simulink model "Parabolic_Shooting_exercise"  (R2020b)
settings: Solver=VariableStepAuto  StartTime=0.0  StopTime=inf  RelTol=1e-3
settings Model: Creator=gbellido  LastModifiedBy=gbellido

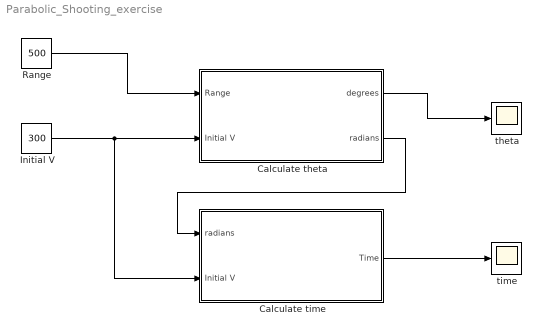
== system Parabolic_Shooting_exercise ==
  Calculate theta : Subsystem
  Calculate time : Subsystem
  Initial V : Constant  Value=300
  Range : Constant  Value=500
  theta : Scope
  time : Scope
  wires:
  Initial V/1 -> Calculate time/2(Initial V), Calculate theta/2(Initial V)
  Calculate theta/1(degrees) -> theta/1
  Calculate time/1(Time) -> time/1
  Calculate theta/2(radians) -> Calculate time/1(radians)
  Range/1 -> Calculate theta/1(Range)

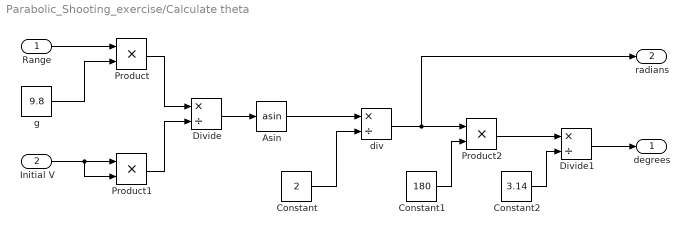
== system Parabolic_Shooting_exercise/Calculate theta ==
  Range : Inport
  Initial V : Inport  Port=2
  Asin : Trigonometry  Operator=asin
  Constant : Constant  Value=2
  Constant1 : Constant  Value=180
  Constant2 : Constant  Value=3.14
  Divide : Product  Inputs=*/
  Divide1 : Product  Inputs=*/
  Product : Product
  Product1 : Product
  Product2 : Product
  div : Product  Inputs=*/
  g : Constant  Value=9.8
  degrees : Outport
  radians : Outport  Port=2
  wires:
  Asin/1 -> div/1
  Divide/1 -> Asin/1
  Product2/1 -> Divide1/1
  Product/1 -> Divide/1
  Constant/1 -> div/2
  Divide1/1 -> degrees/1
  Constant1/1 -> Product2/2
  Product1/1 -> Divide/2
  Constant2/1 -> Divide1/2
  div/1 -> radians/1, Product2/1
  Range/1 -> Product/1
  g/1 -> Product/2
  Initial V/1 -> Product1/2, Product1/1

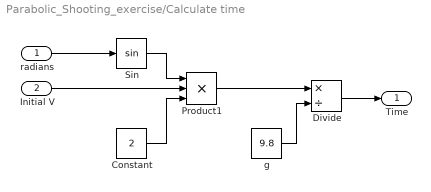
== system Parabolic_Shooting_exercise/Calculate time ==
  radians : Inport
  Initial V : Inport  Port=2
  Constant : Constant  Value=2
  Divide : Product  Inputs=*/
  Product1 : Product  Inputs=3
  Sin : Trigonometry
  g : Constant  Value=9.8
  Time : Outport
  wires:
  Initial V/1 -> Product1/2
  Constant/1 -> Product1/3
  radians/1 -> Sin/1
  Sin/1 -> Product1/1
  Product1/1 -> Divide/1
  g/1 -> Divide/2
  Divide/1 -> Time/1
